simulink model "DiscreteBuck_Offline_Control"  (R2025a)
settings: Solver=FixedStepDiscrete  StartTime=0.0  StopTime=SimTime  FixedStep=Tsim  RelTol=1e-9
undefined symbols (not defined in the file or in its folder): C_buck, Den, DiscIntNeverNeededParam, Iout_buck, k, L_buck, Num, p, R, R1, R2, R3, t1, t2, t2prima, t3, Tsim, Tsw, Vg, Vout_buck, z
libraries: slpidlib x3, spsPWMGeneratorDCDCLib x1
settings Model: Creator=Andres  LastModifiedBy=nelso
settings DataIOCC: SaveFormat=StructureWithTime  ReturnWorkspaceOutputs=off  OutputSaveName=Continuo  SignalLoggingName=ResultDisc

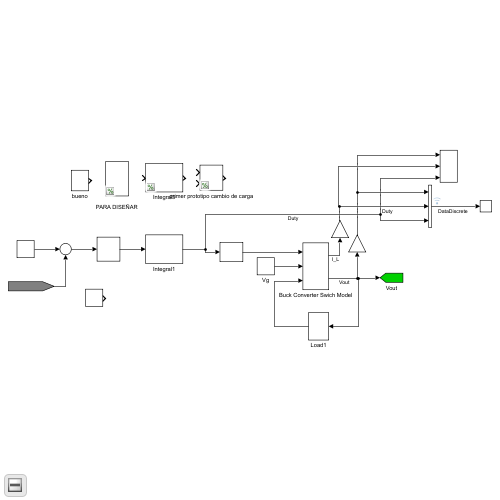
[thumbnail: Simulink's stored preview of the top-level diagram]
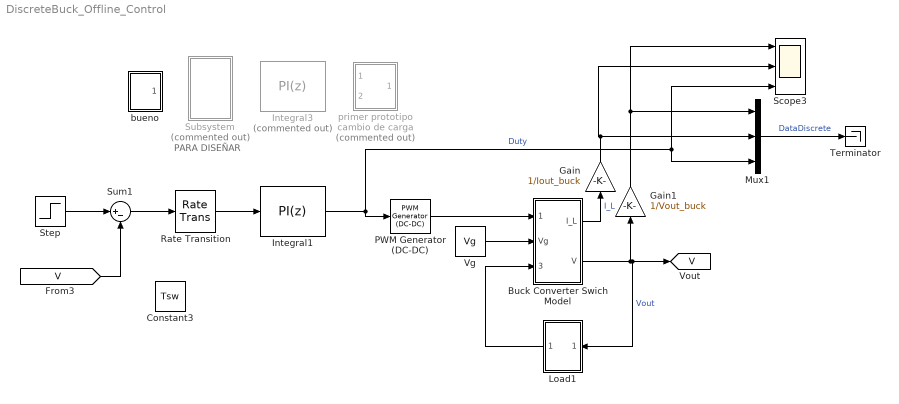
== system DiscreteBuck_Offline_Control ==
  note: PARA DISEÑAR
  Buck Converter Swich Model : Subsystem
      mask Display: image('$imagefile'); % Use "Edit Image" on toolstrip to change.
  Constant3 : Constant  Value=Tsw  SampleTime=Tsw
  Gain : Gain  Gain=1/Iout_buck
  Gain1 : Gain  Gain=1/Vout_buck
  Integral1 : slpidlib/PID Controller  Controller=PI  Form=Parallel  TimeDomain=Discrete-time  UseExternalTs=off  SampleTime=Tsw  IntegratorMethod=Trapezoidal  FilterMethod=Forward Euler  ControllerParametersSource=internal  P=0  I=3.4446  UseKiTs=off  D=1.78707996704397e-06  UseExternalDerivativeSource=off  N=1  UseFilter=off  TunerSelectOption=Transfer Function Based (PID Tuner App)  InitialConditionSource=internal  InitialConditionForIntegrator=0  InitialConditionForFilter=0  DifferentiatorICPrevScaledInput=0  ExternalReset=none  IgnoreLimit=on  TrackingMode=off  Kt=1  LimitOutput=on  SatLimitsSource=internal  UpperSaturationLimit=0.98  LowerSaturationLimit=0  LinearizeAsGain=on  AntiWindupMode=clamping  Kb=1  LimitIntegrator=off  UpperIntegratorSaturationLimit=inf  LowerIntegratorSaturationLimit=-inf  POutMin=[]  POutMax=[]  IOutMin=[]  IOutMax=[]  DOutMin=[]  DOutMax=[]  NOutMin=[]  NOutMax=[]  SumOutMin=[]  SumOutMax=[]  SaturationOutMin=[]  SaturationOutMax=[]  PParamMin=[]  PParamMax=[]  IParamMin=[]  IParamMax=[]  DParamMin=[]  DParamMax=[]  NParamMin=[]  NParamMax=[]  KbParamMin=[]  KbParamMax=[]  KtParamMin=[]  KtParamMax=[]  KbOutMin=[]  KbOutMax=[]  KtOutMin=[]  KtOutMax=[]  IntegratorOutMin=[]  IntegratorOutMax=[]  FilterOutMin=[]  FilterOutMax=[]  SumI1OutMin=[]  SumI1OutMax=[]  SumI2OutMin=[]  SumI2OutMax=[]  SumI3OutMin=[]  SumI3OutMax=[]  SumI4OutMin=[]  SumI4OutMax=[]  SumDOutMin=[]  SumDOutMax=[]  DifferentiatorOutMin=[]  DifferentiatorOutMax=[]  FilterDiffOutCoefMin=[]  FilterDiffOutCoefMax=[]  ReciprocalOutMin=[]  ReciprocalOutMax=[]  SumDenOutMin=[]  SumDenOutMax=[]  SumNumOutMin=[]  SumNumOutMax=[]  DivideOutMin=[]  DivideOutMax=[]  UdiffTsProdOutMin=[]  UdiffTsProdOutMax=[]  NTsProdOutMin=[]  NTsProdOutMax=[]  UintegralTsProdOutMin=[]  UintegralTsProdOutMax=[]  UngainTsProdOutMin=[]  UngainTsProdOutMax=[]  ClampingZeroOutDataTypeStr=Inherit: Inherit via back propagation  ClampingZeroOutMin=[]  ClampingZeroOutMax=[]  FilterDenConstantOutDataTypeStr=Inherit: Inherit via back propagation  FilterDenConstantOutMin=[]  FilterDenConstantOutMax=[]  PCopyOutDataTypeStr=Inherit: Inherit via back propagation  PCopyOutMin=[]  PCopyOutMax=[]  NCopyOutDataTypeStr=Inherit: Inherit via back propagation  NCopyOutMin=[]  NCopyOutMax=[]  IntegratorContinuousStateAttributes=''  IntegratorStateMustResolveToSignalObject=off  IntegratorRTWStateStorageClass=Auto  FilterContinuousStateAttributes=''  FilterStateMustResolveToSignalObject=off  FilterRTWStateStorageClass=Auto  ParallelPVariant=InternalParameters  IdealPVariant=Disabled  IVariant=InternalParameters  DVariant=Disabled  IntegratorVariant=Discrete  SatVariant=Enabled  AWVariant=DiscClampingParallel  PCopyVariant=Disabled  TRVariant=Disabled  FdbkBlocksVariant=Feedback  IdealPFdbkVariant=Passthrough  SatFdbkVariant=Passthrough  DerivativeFilterVariant=Disabled  NVariant=Disabled  NCopyVariant=Disabled_SignalSpec  FilterICVariant=Disabled  IntegratorICVariant=InternalICs  ExternalResetVariant=Disabled  TRSumVariant=Passthrough  SumFdbkVariant=Enabled  SumVariant=Sum_PI  TsampFilterVariant=InternalTs  TsampNgainVariant=Passthrough  TsampIntegralVariant=Disabled_SignalSpec  ExternalSaturationOutDataTypeStr=Inherit: Same as second input  DerivativeSourceVariant=Disabled  PreIntVariant=InternalPreInt
  Integral3 : slpidlib/PID Controller  Commented=on  Controller=PI  Form=Parallel  TimeDomain=Discrete-time  UseExternalTs=off  SampleTime=Tsw  IntegratorMethod=Trapezoidal  FilterMethod=Forward Euler  ControllerParametersSource=internal  P=0.0995683460340593  I=172.683701506663  UseKiTs=off  D=1.78707996704397e-06  UseExternalDerivativeSource=off  N=1  UseFilter=off  TunerSelectOption=Transfer Function Based (PID Tuner App)  InitialConditionSource=internal  InitialConditionForIntegrator=0  InitialConditionForFilter=0  DifferentiatorICPrevScaledInput=0  ExternalReset=none  IgnoreLimit=on  TrackingMode=off  Kt=1  LimitOutput=on  SatLimitsSource=internal  UpperSaturationLimit=0.98  LowerSaturationLimit=0  LinearizeAsGain=on  AntiWindupMode=clamping  Kb=1  LimitIntegrator=off  UpperIntegratorSaturationLimit=inf  LowerIntegratorSaturationLimit=-inf  POutMin=[]  POutMax=[]  IOutMin=[]  IOutMax=[]  DOutMin=[]  DOutMax=[]  NOutMin=[]  NOutMax=[]  SumOutMin=[]  SumOutMax=[]  SaturationOutMin=[]  SaturationOutMax=[]  PParamMin=[]  PParamMax=[]  IParamMin=[]  IParamMax=[]  DParamMin=[]  DParamMax=[]  NParamMin=[]  NParamMax=[]  KbParamMin=[]  KbParamMax=[]  KtParamMin=[]  KtParamMax=[]  KbOutMin=[]  KbOutMax=[]  KtOutMin=[]  KtOutMax=[]  IntegratorOutMin=[]  IntegratorOutMax=[]  FilterOutMin=[]  FilterOutMax=[]  SumI1OutMin=[]  SumI1OutMax=[]  SumI2OutMin=[]  SumI2OutMax=[]  SumI3OutMin=[]  SumI3OutMax=[]  SumI4OutMin=[]  SumI4OutMax=[]  SumDOutMin=[]  SumDOutMax=[]  DifferentiatorOutMin=[]  DifferentiatorOutMax=[]  FilterDiffOutCoefMin=[]  FilterDiffOutCoefMax=[]  ReciprocalOutMin=[]  ReciprocalOutMax=[]  SumDenOutMin=[]  SumDenOutMax=[]  SumNumOutMin=[]  SumNumOutMax=[]  DivideOutMin=[]  DivideOutMax=[]  UdiffTsProdOutMin=[]  UdiffTsProdOutMax=[]  NTsProdOutMin=[]  NTsProdOutMax=[]  UintegralTsProdOutMin=[]  UintegralTsProdOutMax=[]  UngainTsProdOutMin=[]  UngainTsProdOutMax=[]  ClampingZeroOutDataTypeStr=Inherit: Inherit via back propagation  ClampingZeroOutMin=[]  ClampingZeroOutMax=[]  FilterDenConstantOutDataTypeStr=Inherit: Inherit via back propagation  FilterDenConstantOutMin=[]  FilterDenConstantOutMax=[]  PCopyOutDataTypeStr=Inherit: Inherit via back propagation  PCopyOutMin=[]  PCopyOutMax=[]  NCopyOutDataTypeStr=Inherit: Inherit via back propagation  NCopyOutMin=[]  NCopyOutMax=[]  IntegratorContinuousStateAttributes=''  IntegratorStateMustResolveToSignalObject=off  IntegratorRTWStateStorageClass=Auto  FilterContinuousStateAttributes=''  FilterStateMustResolveToSignalObject=off  FilterRTWStateStorageClass=Auto  ParallelPVariant=InternalParameters  IdealPVariant=Disabled  IVariant=InternalParameters  DVariant=Disabled  IntegratorVariant=Discrete  SatVariant=Enabled  AWVariant=DiscClampingParallel  PCopyVariant=Disabled  TRVariant=Disabled  FdbkBlocksVariant=Feedback  IdealPFdbkVariant=Passthrough  SatFdbkVariant=Passthrough  DerivativeFilterVariant=Disabled  NVariant=Disabled  NCopyVariant=Disabled_SignalSpec  FilterICVariant=Disabled  IntegratorICVariant=InternalICs  ExternalResetVariant=Disabled  TRSumVariant=Passthrough  SumFdbkVariant=Enabled  SumVariant=Sum_PI  TsampFilterVariant=InternalTs  TsampNgainVariant=Passthrough  TsampIntegralVariant=Disabled_SignalSpec  ExternalSaturationOutDataTypeStr=Inherit: Same as second input  DerivativeSourceVariant=Disabled  PreIntVariant=InternalPreInt
  Load1 : Subsystem
  Mux1 : Mux  Inputs=3
  PWM Generator (DC-DC) : spsPWMGeneratorDCDCLib/PWM Generator (DC-DC)  Fsw=f_sw  Ts=Tsim
  Rate Transition : RateTransition  OutPortSampleTime=Tsw
  Scope3 : Scope  NumInputPorts=3
      settings: ActiveDisplayYMinimum=-0.14314423307746524  ActiveDisplayYMaximum=1.2882980976971874  YLabel=Voltage (V)
  Step : Step  Time=0.01  After=12
  Subsystem : Subsystem  Commented=on
  Sum1 : Sum  Inputs=|+-
  Terminator : Terminator
  Vg : Constant  Value=Vg  SampleTime=-1
  bueno : Subsystem
  primer prototipo cambio de carga : Subsystem  Commented=on
  tag scope: V=global
  wires:
  Vg/1 -> Buck Converter Swich Model/2(Vg)
  PWM Generator (DC-DC)/1 -> Buck Converter Swich Model/1(PWM)
  Step/1 -> Sum1/1
  [V] -> Sum1/2
  Sum1/1 -> Rate Transition/1
  Buck Converter Swich Model/2(V) -> Gain1/1, Load1/1(Vout), [V]  "Vout"
  Mux1/1 -> Terminator/1  "DataDiscrete"
  Integral1/1 -> PWM Generator (DC-DC)/1, Scope3/3, Mux1/3  "Duty"
  Buck Converter Swich Model/1(I_L) -> Gain/1  "I_L"
  Rate Transition/1 -> Integral1/1
  Load1/1(iload) -> Buck Converter Swich Model/3(I_load)
  Gain/1 -> Scope3/2, Mux1/2
  Gain1/1 -> Scope3/1, Mux1/1

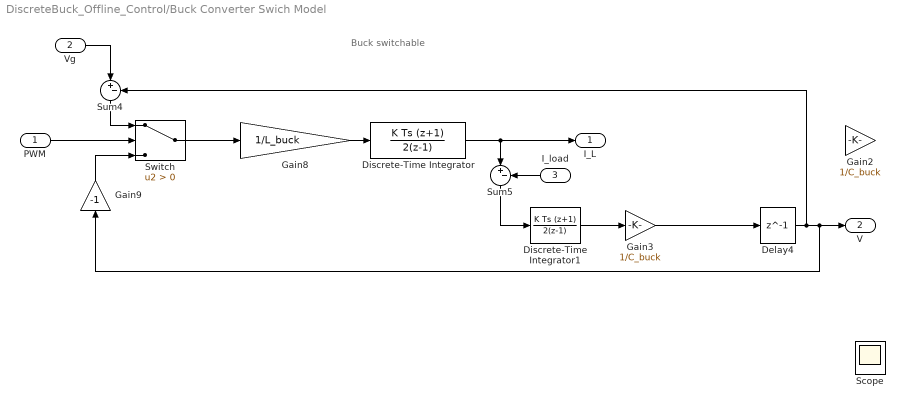
== system DiscreteBuck_Offline_Control/Buck Converter Swich Model ==
  note: Buck switchable
  PWM : Inport
  Vg : Inport  Port=2
  I_load : Inport  Port=3
  Delay4 : Delay  DelayLength=1  InputProcessing=Columns as channels (frame based)
  Discrete-Time Integrator : DiscreteIntegrator  IntegratorMethod=Integration: Trapezoidal  SampleTime=Tsim  LimitOutput=on  LowerSaturationLimit=0  ICPrevOutput=DiscIntNeverNeededParam  ICPrevScaledInput=DiscIntNeverNeededParam
  Discrete-Time Integrator1 : DiscreteIntegrator  IntegratorMethod=Integration: Trapezoidal  SampleTime=Tsim  ICPrevOutput=DiscIntNeverNeededParam  ICPrevScaledInput=DiscIntNeverNeededParam
  Gain2 : Gain  Gain=1/C_buck
  Gain3 : Gain  Gain=1/C_buck
  Gain8 : Gain  Gain=1/L_buck
  Gain9 : Gain  Gain=-1
  Scope : Scope  NumInputPorts=2
      settings: ActiveDisplayYMinimum=-2.4027986803455188  ActiveDisplayYMaximum=21.625188123109673
  Sum4 : Sum  Inputs=|+-
  Sum5 : Sum  Inputs=|+-
  Switch : Switch  Criteria=u2 > Threshold  SaturateOnIntegerOverflow=off  InputSameDT=off
  I_L : Outport
  V : Outport  Port=2
  wires:
  Gain9/1 -> Switch/3
  Switch/1 -> Gain8/1
  Sum4/1 -> Switch/1
  Gain8/1 -> Discrete-Time Integrator/1
  Sum5/1 -> Discrete-Time Integrator1/1
  Discrete-Time Integrator/1 -> I_L/1, Sum5/1
  Vg/1 -> Sum4/1
  I_load/1 -> Sum5/2
  PWM/1 -> Switch/2
  Delay4/1 -> Sum4/2, Gain9/1, V/1
  Discrete-Time Integrator1/1 -> Gain3/1
  Gain3/1 -> Delay4/1

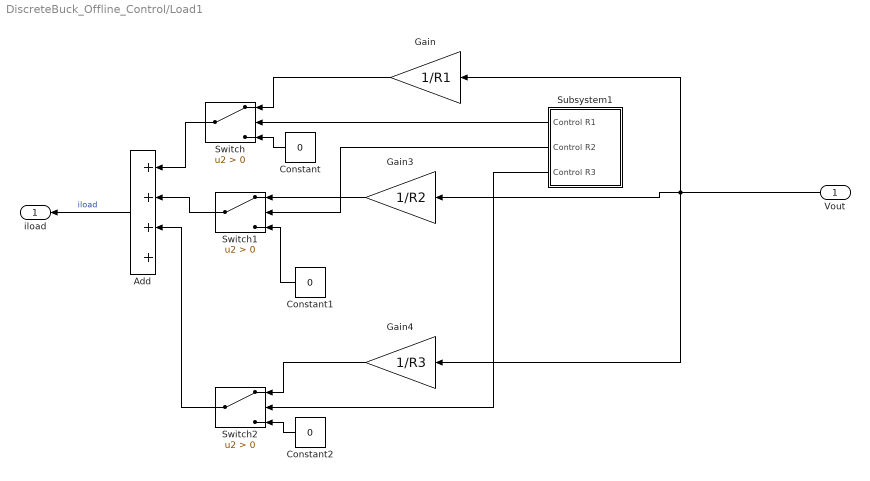
== system DiscreteBuck_Offline_Control/Load1 ==
  Vout : Inport
  Add : Sum  Inputs=++++
  Constant : Constant  Value=0
  Constant1 : Constant  Value=0
  Constant2 : Constant  Value=0
  Gain : Gain  Gain=1/R1
  Gain3 : Gain  Gain=1/R2
  Gain4 : Gain  Gain=1/R3
  Subsystem1 : Subsystem
  Switch : Switch  Criteria=u2 > Threshold  SaturateOnIntegerOverflow=off  InputSameDT=off
  Switch1 : Switch  Criteria=u2 > Threshold  SaturateOnIntegerOverflow=off  InputSameDT=off
  Switch2 : Switch  Criteria=u2 > Threshold  SaturateOnIntegerOverflow=off  InputSameDT=off
  iload : Outport
  wires:
  Add/1 -> iload/1  "iload"
  Gain3/1 -> Switch1/1
  Constant/1 -> Switch/3
  Subsystem1/3(Control R3) -> Switch2/2
  Switch1/1 -> Add/2
  Constant2/1 -> Switch2/3
  Switch/1 -> Add/1
  Vout/1 -> Gain3/1, Gain/1, Gain4/1
  Subsystem1/1(Control R1) -> Switch/2
  Subsystem1/2(Control R2) -> Switch1/2
  Gain/1 -> Switch/1
  Gain4/1 -> Switch2/1
  Switch2/1 -> Add/3
  Constant1/1 -> Switch1/3

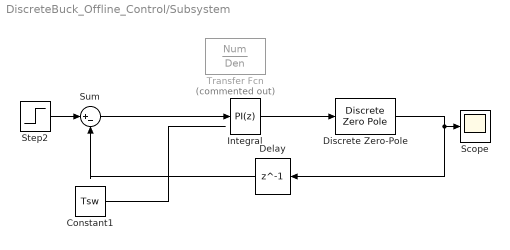
== system DiscreteBuck_Offline_Control/Subsystem ==
  Constant1 : Constant  Value=Tsw
  Delay : Delay  DelayLength=1  InputProcessing=Columns as channels (frame based)
  Discrete Zero-Pole : DiscreteZeroPole  Zeros=z  Poles=p  Gain=k  SampleTime=Tsim
  Integral : slpidlib/PID Controller  Controller=PI  Form=Parallel  TimeDomain=Discrete-time  UseExternalTs=off  SampleTime=Tsw  IntegratorMethod=Trapezoidal  FilterMethod=Forward Euler  ControllerParametersSource=internal  P=0.000518134045814252  I=108.332907969673  UseKiTs=off  D=1.78707996704397e-06  UseExternalDerivativeSource=off  N=1  UseFilter=off  TunerSelectOption=Transfer Function Based (PID Tuner App)  InitialConditionSource=internal  InitialConditionForIntegrator=0  InitialConditionForFilter=0  DifferentiatorICPrevScaledInput=0  ExternalReset=none  IgnoreLimit=on  TrackingMode=off  Kt=1  LimitOutput=on  SatLimitsSource=internal  UpperSaturationLimit=12  LowerSaturationLimit=0  LinearizeAsGain=on  AntiWindupMode=clamping  Kb=1  LimitIntegrator=off  UpperIntegratorSaturationLimit=inf  LowerIntegratorSaturationLimit=-inf  POutMin=[]  POutMax=[]  IOutMin=[]  IOutMax=[]  DOutMin=[]  DOutMax=[]  NOutMin=[]  NOutMax=[]  SumOutMin=[]  SumOutMax=[]  SaturationOutMin=[]  SaturationOutMax=[]  PParamMin=[]  PParamMax=[]  IParamMin=[]  IParamMax=[]  DParamMin=[]  DParamMax=[]  NParamMin=[]  NParamMax=[]  KbParamMin=[]  KbParamMax=[]  KtParamMin=[]  KtParamMax=[]  KbOutMin=[]  KbOutMax=[]  KtOutMin=[]  KtOutMax=[]  IntegratorOutMin=[]  IntegratorOutMax=[]  FilterOutMin=[]  FilterOutMax=[]  SumI1OutMin=[]  SumI1OutMax=[]  SumI2OutMin=[]  SumI2OutMax=[]  SumI3OutMin=[]  SumI3OutMax=[]  SumI4OutMin=[]  SumI4OutMax=[]  SumDOutMin=[]  SumDOutMax=[]  DifferentiatorOutMin=[]  DifferentiatorOutMax=[]  FilterDiffOutCoefMin=[]  FilterDiffOutCoefMax=[]  ReciprocalOutMin=[]  ReciprocalOutMax=[]  SumDenOutMin=[]  SumDenOutMax=[]  SumNumOutMin=[]  SumNumOutMax=[]  DivideOutMin=[]  DivideOutMax=[]  UdiffTsProdOutMin=[]  UdiffTsProdOutMax=[]  NTsProdOutMin=[]  NTsProdOutMax=[]  UintegralTsProdOutMin=[]  UintegralTsProdOutMax=[]  UngainTsProdOutMin=[]  UngainTsProdOutMax=[]  ClampingZeroOutDataTypeStr=Inherit: Inherit via back propagation  ClampingZeroOutMin=[]  ClampingZeroOutMax=[]  FilterDenConstantOutDataTypeStr=Inherit: Inherit via back propagation  FilterDenConstantOutMin=[]  FilterDenConstantOutMax=[]  PCopyOutDataTypeStr=Inherit: Inherit via back propagation  PCopyOutMin=[]  PCopyOutMax=[]  NCopyOutDataTypeStr=Inherit: Inherit via back propagation  NCopyOutMin=[]  NCopyOutMax=[]  IntegratorContinuousStateAttributes=''  IntegratorStateMustResolveToSignalObject=off  IntegratorRTWStateStorageClass=Auto  FilterContinuousStateAttributes=''  FilterStateMustResolveToSignalObject=off  FilterRTWStateStorageClass=Auto  ParallelPVariant=InternalParameters  IdealPVariant=Disabled  IVariant=InternalParameters  DVariant=Disabled  IntegratorVariant=Discrete  SatVariant=Enabled  AWVariant=DiscClampingParallel  PCopyVariant=Disabled  TRVariant=Disabled  FdbkBlocksVariant=Feedback  IdealPFdbkVariant=Passthrough  SatFdbkVariant=Passthrough  DerivativeFilterVariant=Disabled  NVariant=Disabled  NCopyVariant=Disabled_SignalSpec  FilterICVariant=Disabled  IntegratorICVariant=InternalICs  ExternalResetVariant=Disabled  TRSumVariant=Passthrough  SumFdbkVariant=Enabled  SumVariant=Sum_PI  TsampFilterVariant=InternalTs  TsampNgainVariant=Passthrough  TsampIntegralVariant=Disabled_SignalSpec  ExternalSaturationOutDataTypeStr=Inherit: Same as second input  DerivativeSourceVariant=Disabled  PreIntVariant=InternalPreInt
  Scope : Scope
      settings: TimeSpan=0.1  ActiveDisplayYMinimum=-0.625  ActiveDisplayYMaximum=5.625  DataLoggingVariableName=ScopeData2
  Step2 : Step  Time=0  After=5
  Sum : Sum  Inputs=|+-
  Transfer Fcn : TransferFcn  Commented=on  Numerator=Num  Denominator=Den
  wires:
  Constant1/1 -> ?
  Step2/1 -> Sum/1
  Discrete Zero-Pole/1 -> Delay/1, Scope/1
  Delay/1 -> Sum/2
  Sum/1 -> Integral/1
  Integral/1 -> Discrete Zero-Pole/1

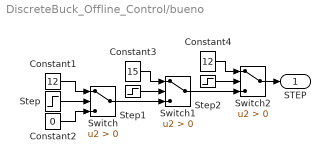
== system DiscreteBuck_Offline_Control/bueno ==
  Constant1 : Constant  Value=12  SampleTime=-1
  Constant2 : Constant  Value=0  SampleTime=-1
  Constant3 : Constant  Value=15  SampleTime=-1
  Constant4 : Constant  Value=12  SampleTime=-1
  Step : Step  Time=0.01
  Step1 : Step  Time=0.03
  Step2 : Step  Time=0.055
  Switch : Switch  Criteria=u2 > Threshold  SaturateOnIntegerOverflow=off  InputSameDT=off
  Switch1 : Switch  Criteria=u2 > Threshold  SaturateOnIntegerOverflow=off  InputSameDT=off
  Switch2 : Switch  Criteria=u2 > Threshold  SaturateOnIntegerOverflow=off  InputSameDT=off
  STEP : Outport
  wires:
  Switch2/1 -> STEP/1
  Constant4/1 -> Switch2/1
  Step2/1 -> Switch2/2
  Switch1/1 -> Switch2/3
  Constant2/1 -> Switch/3
  Step1/1 -> Switch1/2
  Switch/1 -> Switch1/3
  Constant1/1 -> Switch/1
  Constant3/1 -> Switch1/1
  Step/1 -> Switch/2

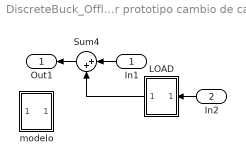
== system DiscreteBuck_Offline_Control/primer prototipo cambio de carga ==
  In1 : Inport
  In2 : Inport  Port=2
  LOAD : Subsystem
  Sum4 : Sum  Inputs=|++
  modelo : Subsystem
  Out1 : Outport
  wires:
  LOAD/1(Out1) -> Sum4/2
  In1/1 -> Sum4/1
  Sum4/1 -> Out1/1
  In2/1 -> LOAD/1(In1)

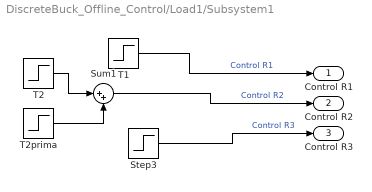
== system DiscreteBuck_Offline_Control/Load1/Subsystem1 ==
  Step3 : Step  Time=t3  SampleTime=0
  Sum1 : Sum  Inputs=|++
  T1 : Step  Time=t1  Before=1  After=0  SampleTime=0
  T2 : Step  Time=t2  SampleTime=0
  T2prima : Step  Time=t2prima  After=-1  SampleTime=0
  Control R1 : Outport
  Control R2 : Outport  Port=2
  Control R3 : Outport  Port=3
  wires:
  Sum1/1 -> Control R2/1  "Control R2"
  T1/1 -> Control R1/1  "Control R1"
  T2prima/1 -> Sum1/2
  T2/1 -> Sum1/1
  Step3/1 -> Control R3/1  "Control R3"

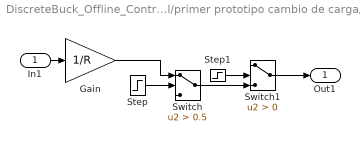
== system DiscreteBuck_Offline_Control/primer prototipo cambio de carga/LOAD ==
  In1 : Inport
  Gain : Gain  Gain=1/R
  Step : Step  Time=0.15  After=-1  SampleTime=Tsim
  Step1 : Step  Time=0.19  SampleTime=Tsim
  Switch : Switch  Criteria=u2 > Threshold  Threshold=0.5  SaturateOnIntegerOverflow=off  InputSameDT=off
  Switch1 : Switch  Criteria=u2 > Threshold  SaturateOnIntegerOverflow=off  InputSameDT=off
  Out1 : Outport
  wires:
  Step/1 -> Switch/2
  Switch/1 -> Switch1/3
  Step1/1 -> Switch1/2
  Switch1/1 -> Out1/1
  In1/1 -> Gain/1
  Gain/1 -> Switch/1

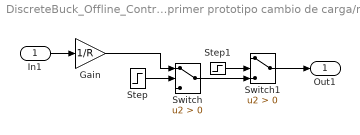
== system DiscreteBuck_Offline_Control/primer prototipo cambio de carga/modelo ==
  In1 : Inport
  Gain : Gain  Gain=1/R
  Step : Step  Time=0.15  SampleTime=Tsim
  Step1 : Step  Time=0.19  SampleTime=Tsim
  Switch : Switch  Criteria=u2 > Threshold  SaturateOnIntegerOverflow=off  InputSameDT=off
  Switch1 : Switch  Criteria=u2 > Threshold  SaturateOnIntegerOverflow=off  InputSameDT=off
  Out1 : Outport
  wires:
  Step/1 -> Switch/2
  Switch/1 -> Switch1/3
  Step1/1 -> Switch1/2
  Switch1/1 -> Out1/1
  In1/1 -> Gain/1
  Gain/1 -> Switch/1
